simulink library "SUB_L4_Task_10ms"  (R2018a)
settings: Solver=VariableStepAuto  StartTime=0.0  StopTime=10.0  RelTol=1e-3
libraries: EmE_MBD_Blockset x75, simulink x11, SUB_L4_Task_10ms_SUB_APTC x1, SUB_L4_Task_10ms_SUB_BRKPEDARB x1, SUB_L4_Task_10ms_SUB_FAULT_MANAGER x1, SUB_L4_Task_10ms_SUB_STATE_CONTROL x1, SUB_L4_Task_10ms_SUB_STEERCTRL x1, simulink_need_slupdate x1
(part 1 of 2)
settings Model: Creator=Chris.Balton  LastModifiedBy=Gavin.Coelho

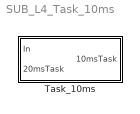
== system SUB_L4_Task_10ms ==
  Task_10ms : Subsystem  TreatAsAtomicUnit=on  SystemSampleTime=0.01

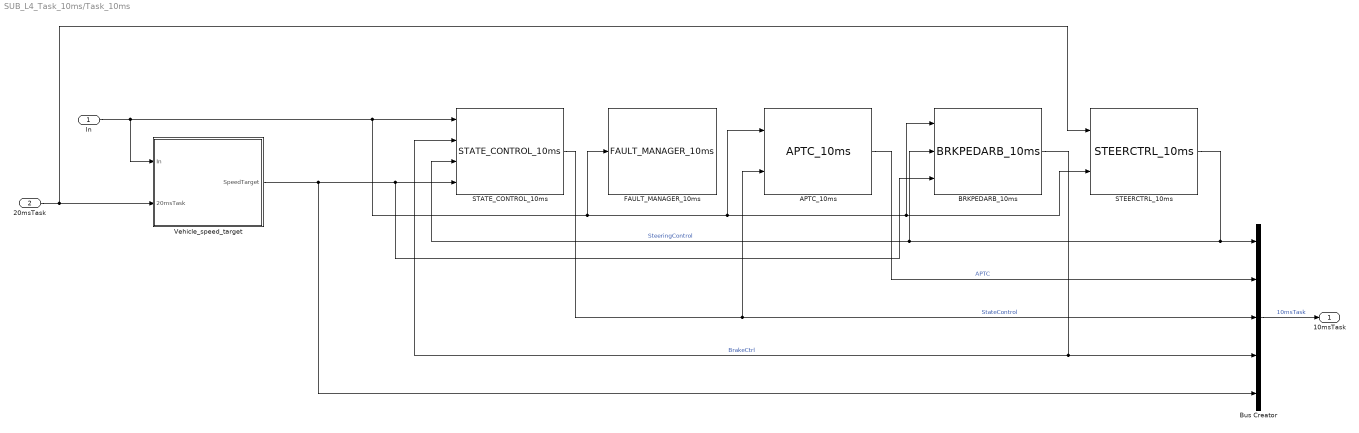
== system SUB_L4_Task_10ms/Task_10ms ==
  In : Inport
  20msTask : Inport  Port=2
  APTC_10ms : SUB_L4_Task_10ms_SUB_APTC/APTC_10ms
  BRKPEDARB_10ms : SUB_L4_Task_10ms_SUB_BRKPEDARB/BRKPEDARB_10ms
  Bus Creator : BusCreator  Inputs=5
  FAULT_MANAGER_10ms : SUB_L4_Task_10ms_SUB_FAULT_MANAGER/FAULT_MANAGER_10ms
  STATE_CONTROL_10ms : SUB_L4_Task_10ms_SUB_STATE_CONTROL/STATE_CONTROL_10ms
  STEERCTRL_10ms : SUB_L4_Task_10ms_SUB_STEERCTRL/STEERCTRL_10ms
  Vehicle_speed_target : Subsystem
  10msTask : Outport
  wires:
  Vehicle_speed_target/1(SpeedTarget) -> BRKPEDARB_10ms/3, STATE_CONTROL_10ms/4, Bus Creator/5
  20msTask/1 -> Vehicle_speed_target/2(20msTask), STEERCTRL_10ms/1
  BRKPEDARB_10ms/1 -> Bus Creator/4, STATE_CONTROL_10ms/2  "BrakeCtrl"
  STATE_CONTROL_10ms/1 -> APTC_10ms/2, Bus Creator/3  "StateControl"
  STEERCTRL_10ms/1 -> BRKPEDARB_10ms/2, STATE_CONTROL_10ms/3, Bus Creator/1  "SteeringControl"
  Bus Creator/1 -> 10msTask/1  "10msTask"
  APTC_10ms/1 -> Bus Creator/2  "APTC"
  In/1 -> Vehicle_speed_target/1(In), STATE_CONTROL_10ms/1, FAULT_MANAGER_10ms/1, APTC_10ms/1, STEERCTRL_10ms/2, BRKPEDARB_10ms/1

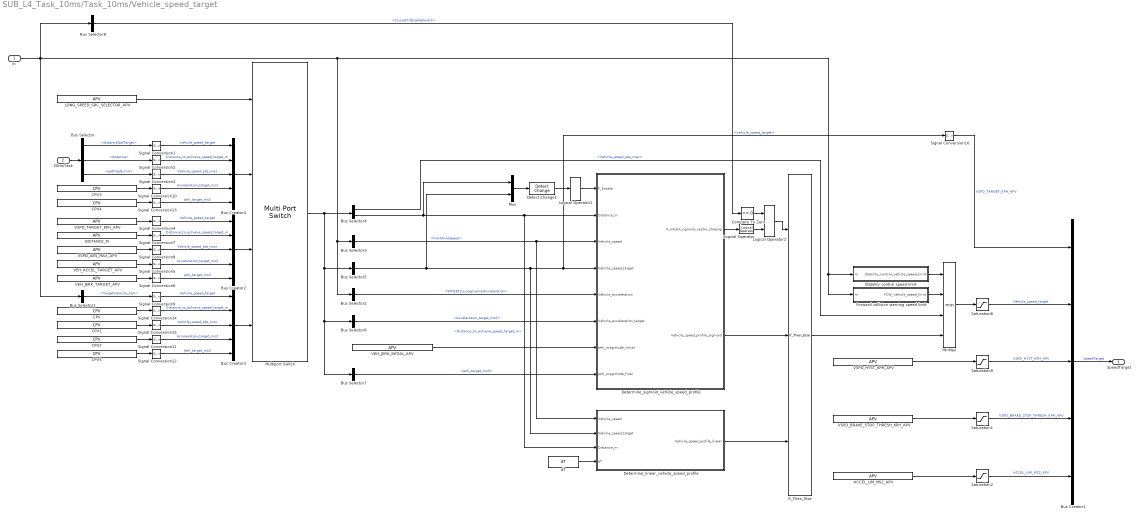
== system SUB_L4_Task_10ms/Task_10ms/Vehicle_speed_target ==
  In : Inport
  20msTask : Inport  Port=2
  ACCEL_LIM_MS2_APV : EmE_MBD_Blockset/Sources/APV  conval=-5
      settings: SourceProductName=PACCAR EmE MBD Blockset
  Bus Creator{1..4} (4 alike) : BusCreator  Inputs=5
  Bus Selector : BusSelector  OutputSignals=mapping.distanceSpdTarget,mapping.distance,mapping.pathSpdLimit
  Bus Selector1 : BusSelector  OutputSignals=PIC_Bus.TargetVelocity_kph
  Bus Selector2 : BusSelector  OutputSignals=CAN.VDC2_0B.SPN1810_LongitudinalAcceleration
  Bus Selector3 : BusSelector  OutputSignals=CAN.EBC2_0B.FrontAxleSpeed
  Bus Selector4 : BusSelector  OutputSignals=Vehicle_speed_abs_max,Distance_to_achieve_speed_target_m
  Bus Selector5 : BusSelector  OutputSignals=Vehicle_speed_target
  Bus Selector6 : BusSelector  OutputSignals=Acceleration_target_ms2
  Bus Selector7 : BusSelector  OutputSignals=Jerk_target_ms3
  Bus Selector8 : BusSelector  OutputSignals=CAN.CCVS_31.CruiseCtrlEnableSwitch
  CPV{,2..4} (4 alike) : EmE_MBD_Blockset/Sources/CPV  conval=0
      settings: SourceProductName=PACCAR EmE MBD Blockset
  CPV1 : EmE_MBD_Blockset/Sources/CPV  conval=255
      settings: SourceProductName=PACCAR EmE MBD Blockset
  CPV5 : EmE_MBD_Blockset/Sources/CPV  conval=0.5
      settings: SourceProductName=PACCAR EmE MBD Blockset
  Compare To Zero : simulink/Logic and Bit Operations/Compare To Zero  relop===  OutDataTypeStr=boolean
  DISTANCE_M : EmE_MBD_Blockset/Sources/APV  conval=DISTANCE_M
      settings: SourceProductName=PACCAR EmE MBD Blockset
  Detect Change1 : simulink/Logic and Bit Operations/Detect Change  vinit=0  InputProcessing=Inherited  OutDataTypeStr=boolean
      settings: AttributesFormatString=IC: %<vinit>
  Determine_linear_vehicle_speed_profile : Subsystem
  Determine_sigmoid_vehicle_speed_profile : Subsystem
  Forward collision warning speed limit : Subsystem
  If_Then_Else : EmE_MBD_Blockset/Signal Routing/If_Then_Else
      settings: SourceProductName=PACCAR EmE MBD Blockset
  LONG_SPEED_SRC_SELECTOR_APV : EmE_MBD_Blockset/Sources/APV  conval=LONG_SPEED_SRC_SELECTOR_APV
      settings: SourceProductName=PACCAR EmE MBD Blockset
  Logical Operator : EmE_MBD_Blockset/Logic and Bit Operations/Logical Operator  Operator=NOT  Inputs=2
      settings: SourceProductName=PACCAR EmE MBD Blockset
  Logical Operator1 : EmE_MBD_Blockset/Logic and Bit Operations/Logical Operator  Operator=OR  Inputs=1
      settings: SourceProductName=PACCAR EmE MBD Blockset
  Logical Operator2 : EmE_MBD_Blockset/Logic and Bit Operations/Logical Operator  Operator=AND  Inputs=2
      settings: SourceProductName=PACCAR EmE MBD Blockset
  MinMax : MinMax  Inputs=4  InputSameDT=on
  Multiport Switch : MultiPortSwitch  DataPortOrder=Specify indices  DataPortIndices={ENUM_LONG_SPEED_DEMAND_SOURCE_T.GPS_PATH,ENUM_LONG_SPEED_DEMAND_SOURCE_T.OVERRIDE,ENUM_LONG_SPEED_DEMAND_SOURCE_T.RW_WAYPOINTS}  DiagnosticForDefault=None
  Mux : Mux  Inputs=2
  Saturation1 : Saturate  UpperLimit=5  LowerLimit=0
      settings: AttributesFormatString=|
      | Min: %<LowerLimit>
      | Max: %<UpperLimit>
  Saturation2 : Saturate  UpperLimit=15.562  LowerLimit=-15.562
      settings: AttributesFormatString=|
      | Min: %<LowerLimit>
      | Max: %<UpperLimit>
  Saturation8 : Saturate  UpperLimit=100  LowerLimit=0
      settings: AttributesFormatString=|
      | Min: %<LowerLimit>
      | Max: %<UpperLimit>
  Saturation9 : Saturate  UpperLimit=5  LowerLimit=0
      settings: AttributesFormatString=|
      | Min: %<LowerLimit>
      | Max: %<UpperLimit>
  Signal Conversion{1..16} (16 alike) : SignalConversion  OverrideOpt=off
  Stability control speed limit : Subsystem
  VEH_ACCEL_TARGET_APV : EmE_MBD_Blockset/Sources/APV  conval=-0.5
      settings: SourceProductName=PACCAR EmE MBD Blockset
  VEH_JERK_INITIAL_APV : EmE_MBD_Blockset/Sources/APV  conval=0.4
      settings: SourceProductName=PACCAR EmE MBD Blockset
  VEH_JERK_TARGET_APV : EmE_MBD_Blockset/Sources/APV  conval=0.2
      settings: SourceProductName=PACCAR EmE MBD Blockset
  VSPD_ABS_MAX_APV : EmE_MBD_Blockset/Sources/APV  conval=255
      settings: SourceProductName=PACCAR EmE MBD Blockset
  VSPD_BRAKE_STOP_THRESH_KPH_APV : EmE_MBD_Blockset/Sources/APV  conval=2
      settings: SourceProductName=PACCAR EmE MBD Blockset
  VSPD_HYST_KPH_APV : EmE_MBD_Blockset/Sources/APV  conval=1
      settings: SourceProductName=PACCAR EmE MBD Blockset
  VSPD_TARGET_KPH_APV : EmE_MBD_Blockset/Sources/APV  conval=VSPD_TARGET_KPH_APV
      settings: SourceProductName=PACCAR EmE MBD Blockset
  dT : EmE_MBD_Blockset/Sources/dT
      settings: SourceProductName=PACCAR EmE MBD Blockset
  SpeedTarget : Outport
  wires:
  Signal Conversion16/1 -> Bus Creator1/1  "VSPD_TARGET_KPH_APV"
  Compare To Zero/1 -> Logical Operator2/1
  Bus Selector8/1 -> Compare To Zero/1  "<CruiseCtrlEnableSwitch>"
  Logical Operator2/1 -> If_Then_Else/1
  VEH_JERK_INITIAL_APV/1 -> Determine_sigmoid_vehicle_speed_profile/7(Jerk_magnitude_initial)
  Bus Selector7/1 -> Determine_sigmoid_vehicle_speed_profile/8(Jerk_magnitude_final)  "<Jerk_target_ms3>"
  CPV5/1 -> Signal Conversion12/1
  Signal Conversion12/1 -> Bus Creator3/5  "Jerk_target_ms3"
  Signal Conversion11/1 -> Bus Creator3/4  "Acceleration_target_ms2"
  Signal Conversion9/1 -> Bus Creator3/1  "Vehicle_speed_target"
  Signal Conversion14/1 -> Bus Creator3/2  "Distance_to_achieve_speed_target_m"
  Signal Conversion15/1 -> Bus Creator3/3  "Vehicle_speed_abs_max"
  Bus Creator3/1 -> Multiport Switch/4
  VEH_JERK_TARGET_APV/1 -> Signal Conversion6/1
  VEH_ACCEL_TARGET_APV/1 -> Signal Conversion5/1
  Bus Creator2/1 -> Multiport Switch/3
  Signal Conversion8/1 -> Bus Creator2/3  "Vehicle_speed_abs_max"
  Signal Conversion7/1 -> Bus Creator2/2  "Distance_to_achieve_speed_target_m"
  Signal Conversion4/1 -> Bus Creator2/1  "Vehicle_speed_target"
  Signal Conversion5/1 -> Bus Creator2/4  "Acceleration_target_ms2"
  Signal Conversion6/1 -> Bus Creator2/5  "Jerk_target_ms3"
  Signal Conversion13/1 -> Bus Creator4/5  "Jerk_target_ms3"
  CPV4/1 -> Signal Conversion13/1
  Determine_sigmoid_vehicle_speed_profile/2(Vehicle_speed_profile_sigmoid) -> If_Then_Else/2
  Bus Selector5/1 -> Mux/2, Determine_sigmoid_vehicle_speed_profile/4(Vehicle_speed_target), Signal Conversion16/1, Determine_linear_vehicle_speed_profile/2(Vehicle_speed_target)  "<Vehicle_speed_target>"
  Mux/1 -> Detect Change1/1
  Detect Change1/1 -> Logical Operator1/1
  Forward collision warning speed limit/1(FCW_vehicle_speed_limit) -> MinMax/2
  Bus Selector4/1 -> MinMax/3  "<Vehicle_speed_abs_max>"
  CPV3/1 -> Signal Conversion10/1
  CPV2/1 -> Signal Conversion11/1
  Signal Conversion10/1 -> Bus Creator4/4  "Acceleration_target_ms2"
  Signal Conversion1/1 -> Bus Creator4/1  "Vehicle_speed_target"
  Signal Conversion2/1 -> Bus Creator4/2  "Distance_to_achieve_speed_target_m"
  Signal Conversion3/1 -> Bus Creator4/3  "Vehicle_speed_abs_max"
  Multiport Switch/1 -> Bus Selector4/1, Bus Selector5/1, Bus Selector6/1, Bus Selector7/1
  CPV1/1 -> Signal Conversion15/1
  CPV/1 -> Signal Conversion14/1
  VSPD_ABS_MAX_APV/1 -> Signal Conversion8/1
  Bus Selector/3 -> Signal Conversion3/1  "<pathSpdLimit>"
  Bus Selector/1 -> Signal Conversion1/1  "<distanceSpdTarget>"
  DISTANCE_M/1 -> Signal Conversion7/1
  VSPD_TARGET_KPH_APV/1 -> Signal Conversion4/1
  Bus Creator4/1 -> Multiport Switch/2
  If_Then_Else/1 -> MinMax/4
  20msTask/1 -> Bus Selector/1
  Bus Selector/2 -> Signal Conversion2/1  "<distance>"
  Bus Selector6/1 -> Determine_sigmoid_vehicle_speed_profile/6(Vehicle_acceleration_target)  "<Acceleration_target_ms2>"
  Logical Operator/1 -> Logical Operator2/2
  Bus Selector4/2 -> Mux/1, Determine_linear_vehicle_speed_profile/3(Distance_m), Determine_sigmoid_vehicle_speed_profile/2(Distance_m)  "<Distance_to_achieve_speed_target_m>"
  Bus Selector3/1 -> Determine_linear_vehicle_speed_profile/1(Vehicle_speed), Determine_sigmoid_vehicle_speed_profile/3(Vehicle_speed)  "<FrontAxleSpeed>"
  Logical Operator1/1 -> Determine_sigmoid_vehicle_speed_profile/1(F_Enable)
  dT/1 -> Determine_linear_vehicle_speed_profile/4(dT)
  Bus Selector2/1 -> Determine_sigmoid_vehicle_speed_profile/5(Vehicle_acceleration)  "<SPN1810_LongitudinalAcceleration>"
  Determine_sigmoid_vehicle_speed_profile/1(F_Inhibit_sigmoid_vector_shaping) -> Logical Operator/1
  Determine_linear_vehicle_speed_profile/1(Vehicle_speed_profile_linear) -> If_Then_Else/3
  Bus Creator1/1 -> SpeedTarget/1  "SpeedTarget"
  Saturation9/1 -> Bus Creator1/3  "VSPD_HYST_KPH_APV"
  Saturation2/1 -> Bus Creator1/5  "ACCEL_LIM_MS2_APV"
  Bus Selector1/1 -> Signal Conversion9/1  "<TargetVelocity_kph>"
  ACCEL_LIM_MS2_APV/1 -> Saturation2/1
  VSPD_BRAKE_STOP_THRESH_KPH_APV/1 -> Saturation1/1
  MinMax/1 -> Saturation8/1
  Saturation1/1 -> Bus Creator1/4  "VSPD_BRAKE_STOP_THRESH_KPH_APV"
  LONG_SPEED_SRC_SELECTOR_APV/1 -> Multiport Switch/1
  Stability control speed limit/1(Stability_control_vehicle_speed_limit) -> MinMax/1
  Saturation8/1 -> Bus Creator1/2  "Vehicle_speed_target"
  VSPD_HYST_KPH_APV/1 -> Saturation9/1
  In/1 -> Bus Selector8/1, Forward collision warning speed limit/1(In), Stability control speed limit/1(In), Bus Selector3/1, Bus Selector2/1, Bus Selector1/1

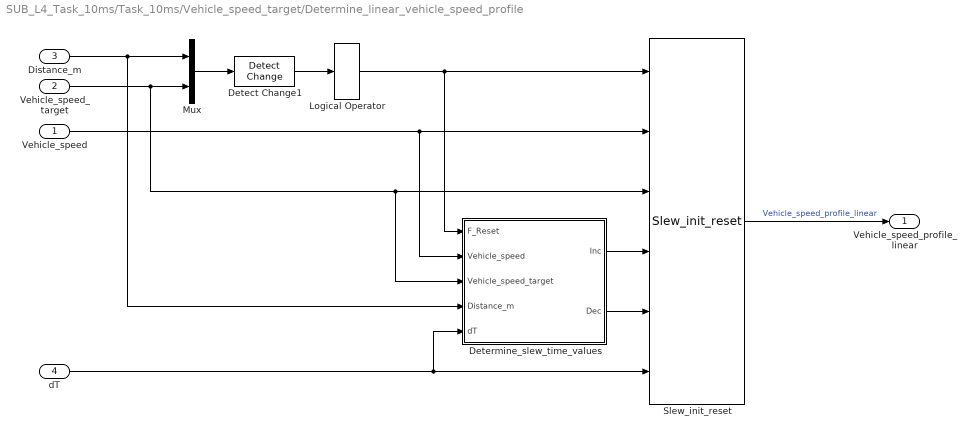
== system SUB_L4_Task_10ms/Task_10ms/Vehicle_speed_target/Determine_linear_vehicle_speed_profile ==
  Vehicle_speed : Inport
  Vehicle_speed_target : Inport  Port=2
  Distance_m : Inport  Port=3
  dT : Inport  Port=4
  Detect Change1 : simulink/Logic and Bit Operations/Detect Change  vinit=0  InputProcessing=Inherited  OutDataTypeStr=boolean
      settings: AttributesFormatString=IC: %<vinit>
  Determine_slew_time_values : Subsystem
  Logical Operator : EmE_MBD_Blockset/Logic and Bit Operations/Logical Operator  Operator=OR  Inputs=1
      settings: SourceProductName=PACCAR EmE MBD Blockset
  Mux : Mux  Inputs=2
  Slew_init_reset : EmE_MBD_Blockset/Math Operators/Slew_init_reset
      settings: SourceProductName=PACCAR EmE MBD Blockset
  Vehicle_speed_profile_linear : Outport  OutputWhenDisabled=reset
  wires:
  Determine_slew_time_values/2(Dec) -> Slew_init_reset/5
  Determine_slew_time_values/1(Inc) -> Slew_init_reset/4
  Vehicle_speed/1 -> Slew_init_reset/2, Determine_slew_time_values/2(Vehicle_speed)
  Distance_m/1 -> Mux/1, Determine_slew_time_values/4(Distance_m)
  Vehicle_speed_target/1 -> Mux/2, Slew_init_reset/3, Determine_slew_time_values/3(Vehicle_speed_target)
  Logical Operator/1 -> Slew_init_reset/1, Determine_slew_time_values/1(F_Reset)
  Mux/1 -> Detect Change1/1
  Detect Change1/1 -> Logical Operator/1
  Slew_init_reset/1 -> Vehicle_speed_profile_linear/1  "Vehicle_speed_profile_linear"
  dT/1 -> Determine_slew_time_values/5(dT), Slew_init_reset/6

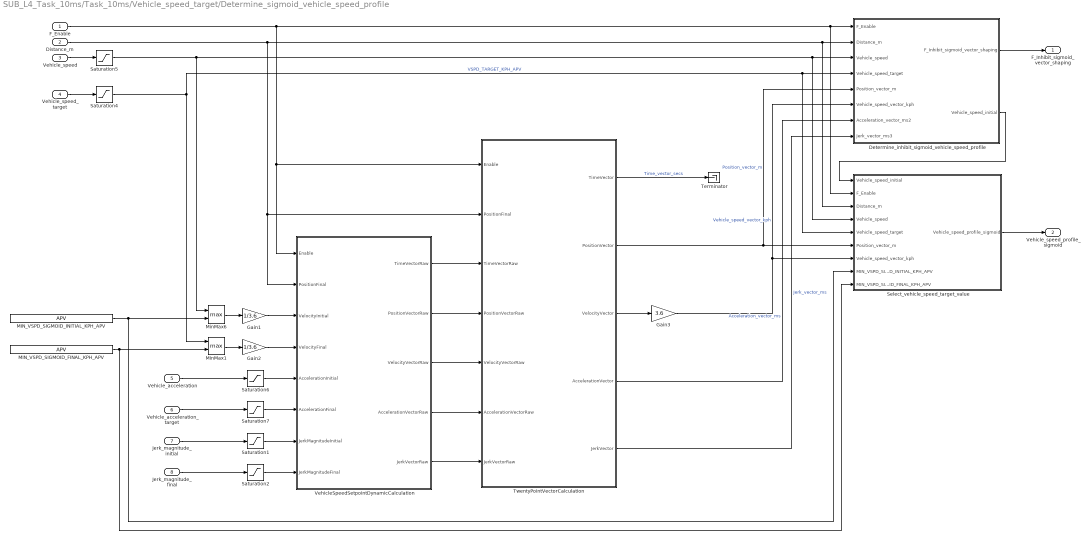
== system SUB_L4_Task_10ms/Task_10ms/Vehicle_speed_target/Determine_sigmoid_vehicle_speed_profile ==
  F_Enable : Inport
  Distance_m : Inport  Port=2
  Vehicle_speed : Inport  Port=3
  Vehicle_speed_target : Inport  Port=4
  Vehicle_acceleration : Inport  Port=5
  Vehicle_acceleration_target : Inport  Port=6
  Jerk_magnitude_initial : Inport  Port=7
  Jerk_magnitude_final : Inport  Port=8
  Determine_inhibit_sigmoid_vehicle_speed_profile : Subsystem
  Gain1 : Gain  Gain=1/3.6
  Gain2 : Gain  Gain=1/3.6
  Gain3 : Gain  Gain=3.6
  MIN_VSPD_SIGMOID_FINAL_KPH_APV : EmE_MBD_Blockset/Sources/APV  conval=0
      settings: SourceProductName=PACCAR EmE MBD Blockset
  MIN_VSPD_SIGMOID_INITIAL_KPH_APV : EmE_MBD_Blockset/Sources/APV  conval=5
      settings: SourceProductName=PACCAR EmE MBD Blockset
  MinMax1 : MinMax  Function=max  Inputs=2  InputSameDT=on
  MinMax6 : MinMax  Function=max  Inputs=2  InputSameDT=on
  Saturation1 : Saturate  UpperLimit=10  LowerLimit=0.001
      settings: AttributesFormatString=|
      | Min: %<LowerLimit>
      | Max: %<UpperLimit>
  Saturation2 : Saturate  UpperLimit=10  LowerLimit=0.001
      settings: AttributesFormatString=|
      | Min: %<LowerLimit>
      | Max: %<UpperLimit>
  Saturation4 : Saturate  UpperLimit=255  LowerLimit=0
      settings: AttributesFormatString=|
      | Min: %<LowerLimit>
      | Max: %<UpperLimit>
  Saturation5 : Saturate  UpperLimit=255  LowerLimit=0
      settings: AttributesFormatString=|
      | Min: %<LowerLimit>
      | Max: %<UpperLimit>
  Saturation6 : Saturate  UpperLimit=15.562  LowerLimit=-15.562
      settings: AttributesFormatString=|
      | Min: %<LowerLimit>
      | Max: %<UpperLimit>
  Saturation7 : Saturate  UpperLimit=15.562  LowerLimit=-15.562
      settings: AttributesFormatString=|
      | Min: %<LowerLimit>
      | Max: %<UpperLimit>
  Select_vehicle_speed_target_value : Subsystem
  Terminator : Terminator
  TwentyPointVectorCalculation : Stateflow chart  TreatAsAtomicUnit=on
  VehicleSpeedSetpointDynamicCalculation : Stateflow chart  TreatAsAtomicUnit=on
  F_Inhibit_sigmoid_vector_shaping : Outport  LibraryBlock=EmE_MBD_Blockset/Sinks/Out  OutputWhenDisabled=reset
  Vehicle_speed_profile_sigmoid : Outport  Port=2
  wires:
  F_Enable/1 -> VehicleSpeedSetpointDynamicCalculation/1(Enable), TwentyPointVectorCalculation/1(Enable), Select_vehicle_speed_target_value/2(F_Enable), Determine_inhibit_sigmoid_vehicle_speed_profile/1(F_Enable)
  Distance_m/1 -> VehicleSpeedSetpointDynamicCalculation/2(PositionFinal), TwentyPointVectorCalculation/2(PositionFinal), Select_vehicle_speed_target_value/3(Distance_m), Determine_inhibit_sigmoid_vehicle_speed_profile/2(Distance_m)
  Gain2/1 -> VehicleSpeedSetpointDynamicCalculation/4(VelocityFinal)
  Gain1/1 -> VehicleSpeedSetpointDynamicCalculation/3(VelocityInitial)
  Vehicle_acceleration/1 -> Saturation6/1
  Gain3/1 -> Determine_inhibit_sigmoid_vehicle_speed_profile/6(Vehicle_speed_vector_kph), Select_vehicle_speed_target_value/7(Vehicle_speed_vector_kph)  "Vehicle_speed_vector_kph"
  Vehicle_acceleration_target/1 -> Saturation7/1
  Determine_inhibit_sigmoid_vehicle_speed_profile/1(F_Inhibit_sigmoid_vector_shaping) -> F_Inhibit_sigmoid_vector_shaping/1
  Vehicle_speed/1 -> Saturation5/1
  Select_vehicle_speed_target_value/1(Vehicle_speed_profile_sigmoid) -> Vehicle_speed_profile_sigmoid/1
  VehicleSpeedSetpointDynamicCalculation/5(JerkVectorRaw) -> TwentyPointVectorCalculation/7(JerkVectorRaw)
  TwentyPointVectorCalculation/1(TimeVector) -> Terminator/1  "Time_vector_secs"
  TwentyPointVectorCalculation/3(VelocityVector) -> Gain3/1
  VehicleSpeedSetpointDynamicCalculation/4(AccelerationVectorRaw) -> TwentyPointVectorCalculation/6(AccelerationVectorRaw)
  TwentyPointVectorCalculation/4(AccelerationVector) -> Determine_inhibit_sigmoid_vehicle_speed_profile/7(Acceleration_vector_ms2)  "Acceleration_vector_ms"
  VehicleSpeedSetpointDynamicCalculation/2(PositionVectorRaw) -> TwentyPointVectorCalculation/4(PositionVectorRaw)
  TwentyPointVectorCalculation/5(JerkVector) -> Determine_inhibit_sigmoid_vehicle_speed_profile/8(Jerk_vector_ms3)  "Jerk_vector_ms"
  VehicleSpeedSetpointDynamicCalculation/1(TimeVectorRaw) -> TwentyPointVectorCalculation/3(TimeVectorRaw)
  TwentyPointVectorCalculation/2(PositionVector) -> Determine_inhibit_sigmoid_vehicle_speed_profile/5(Position_vector_m), Select_vehicle_speed_target_value/6(Position_vector_m)  "Position_vector_m"
  VehicleSpeedSetpointDynamicCalculation/3(VelocityVectorRaw) -> TwentyPointVectorCalculation/5(VelocityVectorRaw)
  Jerk_magnitude_initial/1 -> Saturation1/1
  Jerk_magnitude_final/1 -> Saturation2/1
  MIN_VSPD_SIGMOID_INITIAL_KPH_APV/1 -> MinMax6/2, Select_vehicle_speed_target_value/8(MIN_VSPD_SIGMOID_INITIAL_KPH_APV)
  MIN_VSPD_SIGMOID_FINAL_KPH_APV/1 -> MinMax1/2, Select_vehicle_speed_target_value/9(MIN_VSPD_SIGMOID_FINAL_KPH_APV)
  MinMax1/1 -> Gain2/1
  MinMax6/1 -> Gain1/1
  Determine_inhibit_sigmoid_vehicle_speed_profile/2(Vehicle_speed_initial) -> Select_vehicle_speed_target_value/1(Vehicle_speed_initial)
  Saturation4/1 -> MinMax1/1, Select_vehicle_speed_target_value/5(Vehicle_speed_target), Determine_inhibit_sigmoid_vehicle_speed_profile/4(Vehicle_speed_target)  "VSPD_TARGET_KPH_APV"
  Saturation5/1 -> MinMax6/1, Select_vehicle_speed_target_value/4(Vehicle_speed), Determine_inhibit_sigmoid_vehicle_speed_profile/3(Vehicle_speed)
  Vehicle_speed_target/1 -> Saturation4/1
  Saturation6/1 -> VehicleSpeedSetpointDynamicCalculation/5(AccelerationInitial)
  Saturation7/1 -> VehicleSpeedSetpointDynamicCalculation/6(AccelerationFinal)
  Saturation1/1 -> VehicleSpeedSetpointDynamicCalculation/7(JerkMagnitudeInitial)
  Saturation2/1 -> VehicleSpeedSetpointDynamicCalculation/8(JerkMagnitudeFinal)

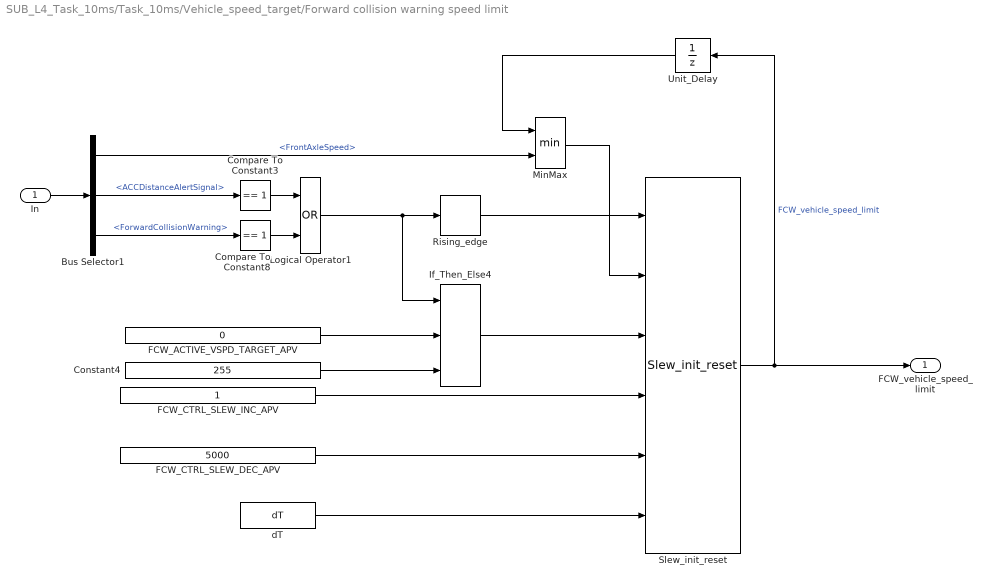
== system SUB_L4_Task_10ms/Task_10ms/Vehicle_speed_target/Forward collision warning speed limit ==
  In : Inport
  Bus Selector1 : BusSelector  OutputSignals=CAN.EBC2_0B.FrontAxleSpeed,CAN.ACC1_2A.ACCDistanceAlertSignal,CAN.ACC1_2A.ForwardCollisionWarning
  Compare To Constant3 : simulink/Logic and Bit Operations/Compare To Constant  relop===  const=1  OutDataTypeStr=boolean
  Compare To Constant8 : simulink/Logic and Bit Operations/Compare To Constant  relop===  const=1  OutDataTypeStr=boolean
  Constant4 : Constant  Value=255
  FCW_ACTIVE_VSPD_TARGET_APV : Constant  Value=0
  FCW_CTRL_SLEW_DEC_APV : Constant  Value=5000
  FCW_CTRL_SLEW_INC_APV : Constant
  If_Then_Else4 : EmE_MBD_Blockset/Signal Routing/If_Then_Else
      settings: SourceProductName=PACCAR EmE MBD Blockset
  Logical Operator1 : Logic  Operator=OR  OutDataTypeStr=boolean
  MinMax : MinMax  Inputs=2  InputSameDT=on
  Rising_edge : EmE_MBD_Blockset/Discontinuities/Rising_edge  initact=off
      settings: AttributesFormatString=Action on IC: %<initact>  SourceProductName=PACCAR EmE MBD Blockset
  Slew_init_reset : EmE_MBD_Blockset/Math Operators/Slew_init_reset
      settings: SourceProductName=PACCAR EmE MBD Blockset
  Unit_Delay : UnitDelay  SampleTime=-1
      settings: AttributesFormatString=IC: %<vinit>
  dT : EmE_MBD_Blockset/Sources/dT
      settings: SourceProductName=PACCAR EmE MBD Blockset
  FCW_vehicle_speed_limit : Outport
  wires:
  MinMax/1 -> Slew_init_reset/2
  FCW_CTRL_SLEW_INC_APV/1 -> Slew_init_reset/4
  FCW_ACTIVE_VSPD_TARGET_APV/1 -> If_Then_Else4/2
  FCW_CTRL_SLEW_DEC_APV/1 -> Slew_init_reset/5
  Slew_init_reset/1 -> Unit_Delay/1, FCW_vehicle_speed_limit/1  "FCW_vehicle_speed_limit"
  Bus Selector1/1 -> MinMax/2  "<FrontAxleSpeed>"
  Constant4/1 -> If_Then_Else4/3
  dT/1 -> Slew_init_reset/6
  Logical Operator1/1 -> Rising_edge/1, If_Then_Else4/1
  If_Then_Else4/1 -> Slew_init_reset/3
  Unit_Delay/1 -> MinMax/1
  Rising_edge/1 -> Slew_init_reset/1
  Bus Selector1/3 -> Compare To Constant8/1  "<ForwardCollisionWarning>"
  Compare To Constant8/1 -> Logical Operator1/2
  Bus Selector1/2 -> Compare To Constant3/1  "<ACCDistanceAlertSignal>"
  Compare To Constant3/1 -> Logical Operator1/1
  In/1 -> Bus Selector1/1

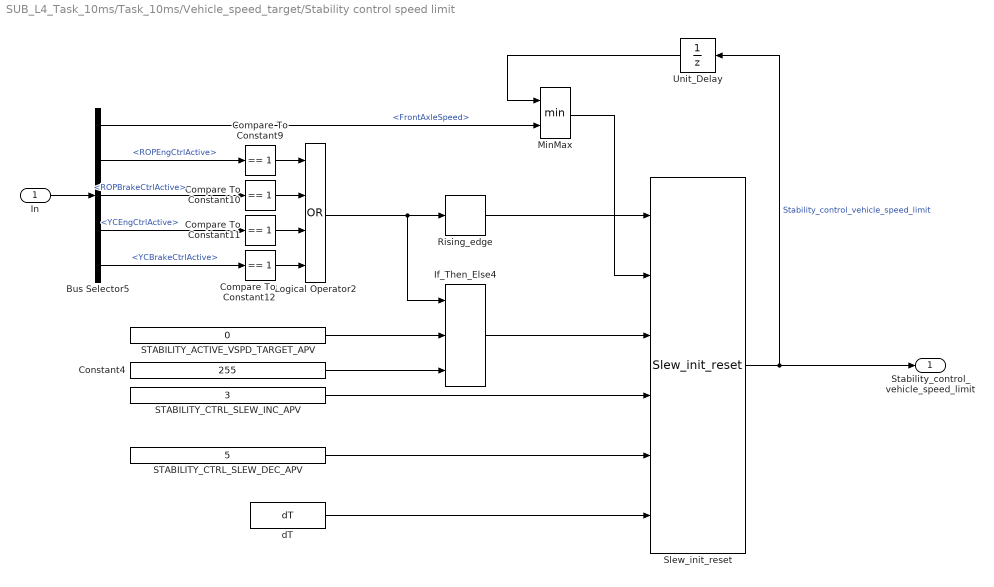
== system SUB_L4_Task_10ms/Task_10ms/Vehicle_speed_target/Stability control speed limit ==
  In : Inport
  Bus Selector5 : BusSelector  OutputSignals=CAN.EBC2_0B.FrontAxleSpeed,CAN.VDC1_0B.ROPEngCtrlActive,CAN.VDC1_0B.ROPBrakeCtrlActive,CAN.VDC1_0B.YCEngCtrlActive,CAN.VDC1_0B.YCBrakeCtrlActive
  Compare To Constant{9..12} (4 alike) : simulink/Logic and Bit Operations/Compare To Constant  relop===  const=1  OutDataTypeStr=boolean
  Constant4 : Constant  Value=255
  If_Then_Else4 : EmE_MBD_Blockset/Signal Routing/If_Then_Else
      settings: SourceProductName=PACCAR EmE MBD Blockset
  Logical Operator2 : Logic  Operator=OR  Inputs=4  OutDataTypeStr=boolean
  MinMax : MinMax  Inputs=2  InputSameDT=on
  Rising_edge : EmE_MBD_Blockset/Discontinuities/Rising_edge  initact=off
      settings: AttributesFormatString=Action on IC: %<initact>  SourceProductName=PACCAR EmE MBD Blockset
  STABILITY_ACTIVE_VSPD_TARGET_APV : Constant  Value=0
  STABILITY_CTRL_SLEW_DEC_APV : Constant  Value=5
  STABILITY_CTRL_SLEW_INC_APV : Constant  Value=3
  Slew_init_reset : EmE_MBD_Blockset/Math Operators/Slew_init_reset
      settings: SourceProductName=PACCAR EmE MBD Blockset
  Unit_Delay : UnitDelay  SampleTime=-1
      settings: AttributesFormatString=IC: %<vinit>
  dT : EmE_MBD_Blockset/Sources/dT
      settings: SourceProductName=PACCAR EmE MBD Blockset
  Stability_control_vehicle_speed_limit : Outport
  wires:
  Unit_Delay/1 -> MinMax/1
  Bus Selector5/1 -> MinMax/2  "<FrontAxleSpeed>"
  MinMax/1 -> Slew_init_reset/2
  Rising_edge/1 -> Slew_init_reset/1
  Slew_init_reset/1 -> Unit_Delay/1, Stability_control_vehicle_speed_limit/1  "Stability_control_vehicle_speed_limit"
  Logical Operator2/1 -> Rising_edge/1, If_Then_Else4/1
  Bus Selector5/3 -> Compare To Constant10/1  "<ROPBrakeCtrlActive>"
  In/1 -> Bus Selector5/1
  If_Then_Else4/1 -> Slew_init_reset/3
  STABILITY_ACTIVE_VSPD_TARGET_APV/1 -> If_Then_Else4/2
  STABILITY_CTRL_SLEW_DEC_APV/1 -> Slew_init_reset/5
  STABILITY_CTRL_SLEW_INC_APV/1 -> Slew_init_reset/4
  Constant4/1 -> If_Then_Else4/3
  dT/1 -> Slew_init_reset/6
  Compare To Constant11/1 -> Logical Operator2/3
  Compare To Constant9/1 -> Logical Operator2/1
  Compare To Constant12/1 -> Logical Operator2/4
  Compare To Constant10/1 -> Logical Operator2/2
  Bus Selector5/5 -> Compare To Constant12/1  "<YCBrakeCtrlActive>"
  Bus Selector5/2 -> Compare To Constant9/1  "<ROPEngCtrlActive>"
  Bus Selector5/4 -> Compare To Constant11/1  "<YCEngCtrlActive>"

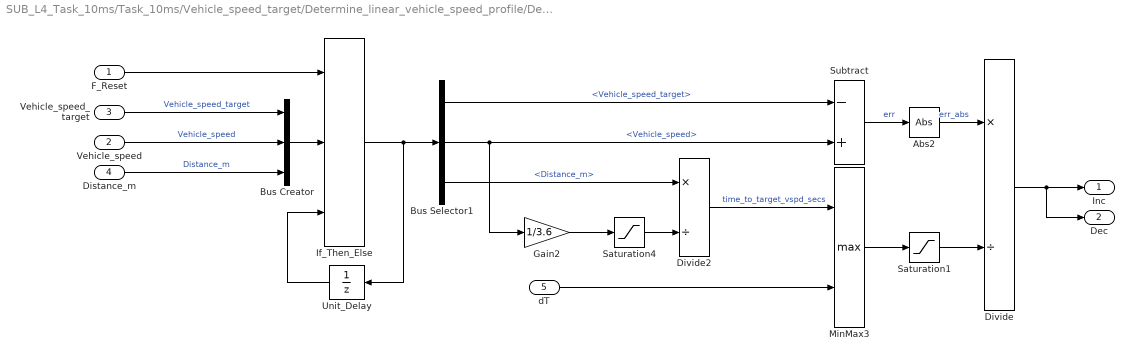
== system SUB_L4_Task_10ms/Task_10ms/Vehicle_speed_target/Determine_linear_vehicle_speed_profile/Determine_slew_time_values ==
  F_Reset : Inport
  Vehicle_speed : Inport  Port=2
  Vehicle_speed_target : Inport  Port=3
  Distance_m : Inport  Port=4
  dT : Inport  Port=5
  Abs2 : EmE_MBD_Blockset/Math Operators/Abs
      settings: SourceProductName=PACCAR EmE MBD Blockset
  Bus Creator : BusCreator  Inputs=3
  Bus Selector1 : BusSelector  OutputSignals=Vehicle_speed_target,Vehicle_speed,Distance_m
  Divide : Product  Inputs=*/  InputSameDT=on
  Divide2 : Product  Inputs=*/  InputSameDT=on
  Gain2 : Gain  Gain=1/3.6
  If_Then_Else : EmE_MBD_Blockset/Signal Routing/If_Then_Else
      settings: SourceProductName=PACCAR EmE MBD Blockset
  MinMax3 : MinMax  Function=max  Inputs=2  InputSameDT=on
  Saturation1 : Saturate  UpperLimit=Inf  LowerLimit=0.001
      settings: AttributesFormatString=|
      | Min: %<LowerLimit>
      | Max: %<UpperLimit>
  Saturation4 : Saturate  UpperLimit=255  LowerLimit=0.001
      settings: AttributesFormatString=|
      | Min: %<LowerLimit>
      | Max: %<UpperLimit>
  Subtract : Sum  Inputs=-+  InputSameDT=on
  Unit_Delay : UnitDelay  SampleTime=-1
      settings: AttributesFormatString=IC: %<vinit>
  Inc : Outport
  Dec : Outport  Port=2
  wires:
  F_Reset/1 -> If_Then_Else/1
  Vehicle_speed/1 -> Bus Creator/2  "Vehicle_speed"
  Vehicle_speed_target/1 -> Bus Creator/1  "Vehicle_speed_target"
  Distance_m/1 -> Bus Creator/3  "Distance_m"
  Unit_Delay/1 -> If_Then_Else/3
  If_Then_Else/1 -> Bus Selector1/1, Unit_Delay/1
  Bus Creator/1 -> If_Then_Else/2
  Saturation1/1 -> Divide/2
  Divide/1 -> Inc/1, Dec/1
  Abs2/1 -> Divide/1  "err_abs"
  MinMax3/1 -> Saturation1/1
  Saturation4/1 -> Divide2/2
  dT/1 -> MinMax3/2
  Bus Selector1/1 -> Subtract/1  "<Vehicle_speed_target>"
  Divide2/1 -> MinMax3/1  "time_to_target_vspd_secs"
  Gain2/1 -> Saturation4/1
  Subtract/1 -> Abs2/1  "err"
  Bus Selector1/3 -> Divide2/1  "<Distance_m>"
  Bus Selector1/2 -> Subtract/2, Gain2/1  "<Vehicle_speed>"

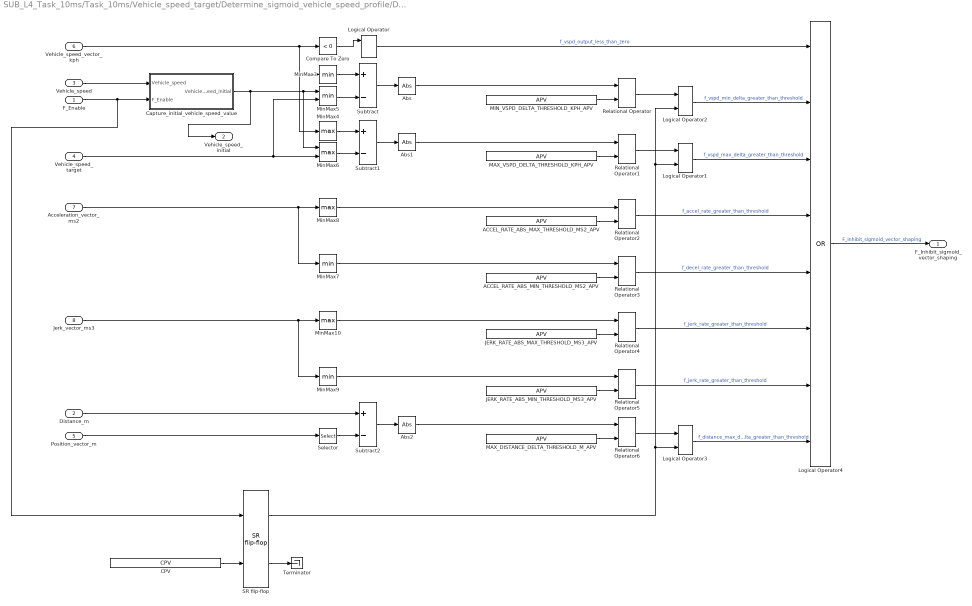
== system SUB_L4_Task_10ms/Task_10ms/Vehicle_speed_target/Determine_sigmoid_vehicle_speed_profile/Determine_inhibit_sigmoid_vehicle_speed_profile ==
  F_Enable : Inport
  Distance_m : Inport  Port=2
  Vehicle_speed : Inport  Port=3
  Vehicle_speed_target : Inport  Port=4
  Position_vector_m : Inport  Port=5
  Vehicle_speed_vector_kph : Inport  Port=6
  Acceleration_vector_ms2 : Inport  Port=7
  Jerk_vector_ms3 : Inport  Port=8
  ACCEL_RATE_ABS_MAX_THRESHOLD_MS2_APV : EmE_MBD_Blockset/Sources/APV  conval=5
      settings: SourceProductName=PACCAR EmE MBD Blockset
  ACCEL_RATE_ABS_MIN_THRESHOLD_MS2_APV : EmE_MBD_Blockset/Sources/APV  conval=-5
      settings: SourceProductName=PACCAR EmE MBD Blockset
  Abs : EmE_MBD_Blockset/Math Operators/Abs
      settings: SourceProductName=PACCAR EmE MBD Blockset
  Abs1 : EmE_MBD_Blockset/Math Operators/Abs
      settings: SourceProductName=PACCAR EmE MBD Blockset
  Abs2 : EmE_MBD_Blockset/Math Operators/Abs
      settings: SourceProductName=PACCAR EmE MBD Blockset
  CPV : EmE_MBD_Blockset/Sources/CPV  conval=false
      settings: SourceProductName=PACCAR EmE MBD Blockset
  Capture_initial_vehicle_speed_value : Subsystem
  Compare To Zero : simulink/Logic and Bit Operations/Compare To Zero  relop=<  OutDataTypeStr=boolean
  JERK_RATE_ABS_MAX_THRESHOLD_MS3_APV : EmE_MBD_Blockset/Sources/APV  conval=5
      settings: SourceProductName=PACCAR EmE MBD Blockset
  JERK_RATE_ABS_MIN_THRESHOLD_MS3_APV : EmE_MBD_Blockset/Sources/APV  conval=-5
      settings: SourceProductName=PACCAR EmE MBD Blockset
  Logical Operator : EmE_MBD_Blockset/Logic and Bit Operations/Logical Operator  Operator=OR  Inputs=1
      settings: SourceProductName=PACCAR EmE MBD Blockset
  Logical Operator1 : EmE_MBD_Blockset/Logic and Bit Operations/Logical Operator  Operator=AND  Inputs=2
      settings: SourceProductName=PACCAR EmE MBD Blockset
  Logical Operator2 : EmE_MBD_Blockset/Logic and Bit Operations/Logical Operator  Operator=AND  Inputs=2
      settings: SourceProductName=PACCAR EmE MBD Blockset
  Logical Operator3 : EmE_MBD_Blockset/Logic and Bit Operations/Logical Operator  Operator=AND  Inputs=2
      settings: SourceProductName=PACCAR EmE MBD Blockset
  Logical Operator4 : Logic  Operator=OR  Inputs=8  AllPortsSameDT=off  OutDataTypeStr=boolean
  MAX_DISTANCE_DELTA_THRESHOLD_M_APV : EmE_MBD_Blockset/Sources/APV  conval=0.5
      settings: SourceProductName=PACCAR EmE MBD Blockset
  MAX_VSPD_DELTA_THRESHOLD_KPH_APV : EmE_MBD_Blockset/Sources/APV  conval=5
      settings: SourceProductName=PACCAR EmE MBD Blockset
  MIN_VSPD_DELTA_THRESHOLD_KPH_APV : EmE_MBD_Blockset/Sources/APV  conval=5
      settings: SourceProductName=PACCAR EmE MBD Blockset
  MinMax10 : MinMax  Function=max  InputSameDT=on
  MinMax3 : MinMax  InputSameDT=on
  MinMax4 : MinMax  Function=max  InputSameDT=on
  MinMax5 : MinMax  Inputs=2  InputSameDT=on
  MinMax6 : MinMax  Function=max  Inputs=2  InputSameDT=on
  MinMax7 : MinMax  InputSameDT=on
  MinMax8 : MinMax  Function=max  InputSameDT=on
  MinMax9 : MinMax  InputSameDT=on
  Relational Operator{,1..2,4,6} (5 alike) : EmE_MBD_Blockset/Logic and Bit Operations/Relational Operator  func=>
      settings: SourceProductName=PACCAR EmE MBD Blockset
  Relational Operator3 : EmE_MBD_Blockset/Logic and Bit Operations/Relational Operator  func=<
      settings: SourceProductName=PACCAR EmE MBD Blockset
  Relational Operator5 : EmE_MBD_Blockset/Logic and Bit Operations/Relational Operator  func=<
      settings: SourceProductName=PACCAR EmE MBD Blockset
  SR flip-flop : EmE_MBD_Blockset/Logic and Bit Operations/SR flip-flop
      settings: SourceProductName=PACCAR EmE MBD Blockset
  Selector : Selector  InputPortWidth=33  IndexOptions=Index vector (dialog)  Indices=33  OutputSizes=1
  Subtract : Sum  Inputs=+-  InputSameDT=on
  Subtract1 : Sum  Inputs=+-  InputSameDT=on
  Subtract2 : Sum  Inputs=+-  InputSameDT=on
  Terminator : Terminator
  F_Inhibit_sigmoid_vector_shaping : Outport  LibraryBlock=EmE_MBD_Blockset/Sinks/Out  OutputWhenDisabled=reset
  Vehicle_speed_initial : Outport  Port=2
  wires:
  Compare To Zero/1 -> Logical Operator/1
  F_Enable/1 -> SR flip-flop/1, Capture_initial_vehicle_speed_value/2(F_Enable)
  ACCEL_RATE_ABS_MIN_THRESHOLD_MS2_APV/1 -> Relational Operator3/2
  Logical Operator4/1 -> F_Inhibit_sigmoid_vector_shaping/1  "F_Inhibit_sigmoid_vector_shaping"
  CPV/1 -> SR flip-flop/2
  Relational Operator4/1 -> Logical Operator4/6  "f_jerk_rate_greater_than_threshold"
  SR flip-flop/2 -> Terminator/1
  MinMax7/1 -> Relational Operator3/1
  SR flip-flop/1 -> Logical Operator3/2, Logical Operator1/2, Logical Operator2/2
  MinMax3/1 -> Subtract/1
  Relational Operator3/1 -> Logical Operator4/5  "f_decel_rate_greater_than_threshold"
  Relational Operator2/1 -> Logical Operator4/4  "f_accel_rate_greater_than_threshold"
  Vehicle_speed_vector_kph/1 -> MinMax4/1, MinMax3/1, Compare To Zero/1
  Acceleration_vector_ms2/1 -> MinMax7/1, MinMax8/1
  JERK_RATE_ABS_MAX_THRESHOLD_MS3_APV/1 -> Relational Operator4/2
  Relational Operator/1 -> Logical Operator2/1
  MinMax8/1 -> Relational Operator2/1
  ACCEL_RATE_ABS_MAX_THRESHOLD_MS2_APV/1 -> Relational Operator2/2
  MinMax10/1 -> Relational Operator4/1
  Relational Operator5/1 -> Logical Operator4/7  "f_jerk_rate_greater_than_threshold"
  Logical Operator1/1 -> Logical Operator4/3  "f_vspd_max_delta_greater_than_threshold"
  Abs/1 -> Relational Operator/1
  Abs1/1 -> Relational Operator1/1
  Jerk_vector_ms3/1 -> MinMax9/1, MinMax10/1
  MIN_VSPD_DELTA_THRESHOLD_KPH_APV/1 -> Relational Operator/2
  MinMax4/1 -> Subtract1/1
  Logical Operator/1 -> Logical Operator4/1  "f_vspd_output_less_than_zero"
  JERK_RATE_ABS_MIN_THRESHOLD_MS3_APV/1 -> Relational Operator5/2
  MinMax9/1 -> Relational Operator5/1
  Logical Operator2/1 -> Logical Operator4/2  "f_vspd_min_delta_greater_than_threshold"
  MAX_VSPD_DELTA_THRESHOLD_KPH_APV/1 -> Relational Operator1/2
  Relational Operator1/1 -> Logical Operator1/1
  Subtract1/1 -> Abs1/1
  Subtract/1 -> Abs/1
  MinMax5/1 -> Subtract/2
  MinMax6/1 -> Subtract1/2
  Vehicle_speed_target/1 -> MinMax5/2, MinMax6/2
  Capture_initial_vehicle_speed_value/1(Vehicle_speed_initial) -> Vehicle_speed_initial/1, MinMax6/1, MinMax5/1
  Vehicle_speed/1 -> Capture_initial_vehicle_speed_value/1(Vehicle_speed)
  MAX_DISTANCE_DELTA_THRESHOLD_M_APV/1 -> Relational Operator6/2
  Abs2/1 -> Relational Operator6/1
  Subtract2/1 -> Abs2/1
  Distance_m/1 -> Subtract2/1
  Logical Operator3/1 -> Logical Operator4/8  "f_distance_max_delta_greater_than_threshold"
  Selector/1 -> Subtract2/2
  Position_vector_m/1 -> Selector/1
  Relational Operator6/1 -> Logical Operator3/1

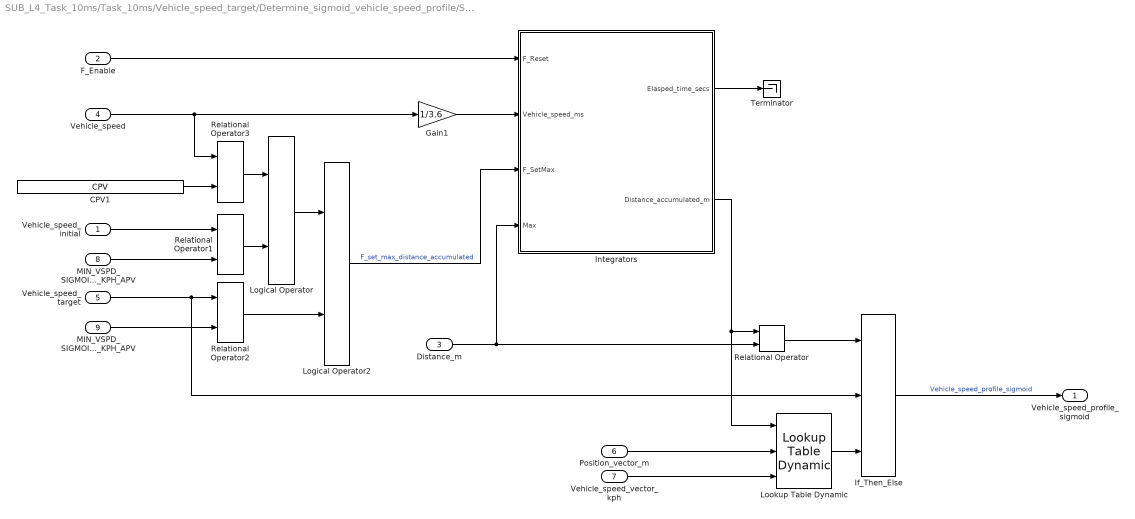
== system SUB_L4_Task_10ms/Task_10ms/Vehicle_speed_target/Determine_sigmoid_vehicle_speed_profile/Select_vehicle_speed_target_value ==
  Vehicle_speed_initial : Inport
  F_Enable : Inport  Port=2
  Distance_m : Inport  Port=3
  Vehicle_speed : Inport  Port=4
  Vehicle_speed_target : Inport  Port=5
  Position_vector_m : Inport  Port=6
  Vehicle_speed_vector_kph : Inport  Port=7
  MIN_VSPD_SIGMOID_INITIAL_KPH_APV : Inport  Port=8
  MIN_VSPD_SIGMOID_FINAL_KPH_APV : Inport  Port=9
  CPV1 : EmE_MBD_Blockset/Sources/CPV  conval=0.1
      settings: SourceProductName=PACCAR EmE MBD Blockset
  Gain1 : Gain  Gain=1/3.6
  If_Then_Else : EmE_MBD_Blockset/Signal Routing/If_Then_Else
      settings: SourceProductName=PACCAR EmE MBD Blockset
  Integrators : Subsystem
  Logical Operator : EmE_MBD_Blockset/Logic and Bit Operations/Logical Operator  Operator=OR  Inputs=2
      settings: SourceProductName=PACCAR EmE MBD Blockset
  Logical Operator2 : EmE_MBD_Blockset/Logic and Bit Operations/Logical Operator  Operator=AND  Inputs=2
      settings: SourceProductName=PACCAR EmE MBD Blockset
  Lookup Table Dynamic : simulink/Lookup Tables/Lookup Table Dynamic  LookUpMeth=Interpolation-Use End Values  OutDataType=fixdt('double')  OutScaling=[]  OutputDataTypeScalingMode=Specify via dialog  OutDataTypeStr=double  DoSatur=off
      settings: SourceProductName=Simulink
  Relational Operator : EmE_MBD_Blockset/Logic and Bit Operations/Relational Operator  func===
      settings: SourceProductName=PACCAR EmE MBD Blockset
  Relational Operator1 : EmE_MBD_Blockset/Logic and Bit Operations/Relational Operator  func=<
      settings: SourceProductName=PACCAR EmE MBD Blockset
  Relational Operator2 : EmE_MBD_Blockset/Logic and Bit Operations/Relational Operator  func=<
      settings: SourceProductName=PACCAR EmE MBD Blockset
  Relational Operator3 : EmE_MBD_Blockset/Logic and Bit Operations/Relational Operator  func=<
      settings: SourceProductName=PACCAR EmE MBD Blockset
  Terminator : Terminator
  Vehicle_speed_profile_sigmoid : Outport
  wires:
  Vehicle_speed_target/1 -> If_Then_Else/2, Relational Operator2/1
  If_Then_Else/1 -> Vehicle_speed_profile_sigmoid/1  "Vehicle_speed_profile_sigmoid"
  Distance_m/1 -> Relational Operator/2, Integrators/4(Max)
  Vehicle_speed/1 -> Relational Operator3/1, Gain1/1
  Position_vector_m/1 -> Lookup Table Dynamic/2
  Integrators/1(Elasped_time_secs) -> Terminator/1
  Vehicle_speed_vector_kph/1 -> Lookup Table Dynamic/3
  Lookup Table Dynamic/1 -> If_Then_Else/3
  F_Enable/1 -> Integrators/1(F_Reset)
  Vehicle_speed_initial/1 -> Relational Operator1/1
  Relational Operator2/1 -> Logical Operator2/2
  MIN_VSPD_SIGMOID_INITIAL_KPH_APV/1 -> Relational Operator1/2
  MIN_VSPD_SIGMOID_FINAL_KPH_APV/1 -> Relational Operator2/2
  Integrators/2(Distance_accumulated_m) -> Lookup Table Dynamic/1, Relational Operator/1
  Gain1/1 -> Integrators/2(Vehicle_speed_ms)
  Relational Operator/1 -> If_Then_Else/1
  Relational Operator3/1 -> Logical Operator/1
  Logical Operator/1 -> Logical Operator2/1
  Relational Operator1/1 -> Logical Operator/2
  CPV1/1 -> Relational Operator3/2
  Logical Operator2/1 -> Integrators/3(F_SetMax)  "F_set_max_distance_accumulated"

== system SUB_L4_Task_10ms/Task_10ms/Vehicle_speed_target/Determine_sigmoid_vehicle_speed_profile/Determine_inhibit_sigmoid_vehicle_speed_profile/Capture_initial_vehicle_speed_value ==
  Vehicle_speed : Inport
  F_Enable : Inport  Port=2
  If_Then_Else : EmE_MBD_Blockset/Signal Routing/If_Then_Else
      settings: SourceProductName=PACCAR EmE MBD Blockset
  Unit_Delay : UnitDelay  SampleTime=-1
      settings: AttributesFormatString=IC: %<vinit>
  Vehicle_speed_initial : Outport
  wires:
  If_Then_Else/1 -> Unit_Delay/1, Vehicle_speed_initial/1  "Vehicle_speed_initial"
  F_Enable/1 -> If_Then_Else/1
  Unit_Delay/1 -> If_Then_Else/3
  Vehicle_speed/1 -> If_Then_Else/2

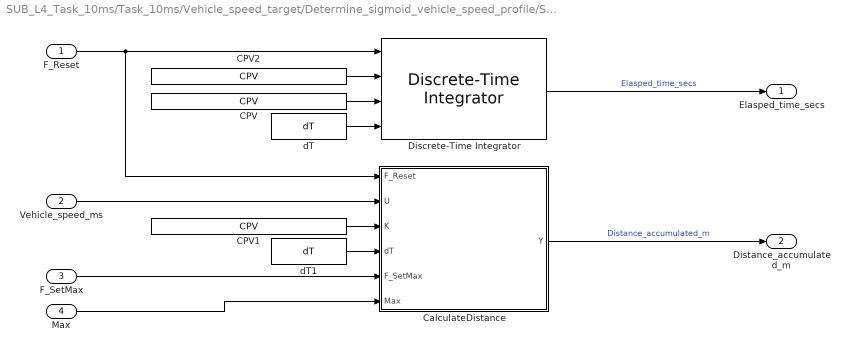
== system SUB_L4_Task_10ms/Task_10ms/Vehicle_speed_target/Determine_sigmoid_vehicle_speed_profile/Select_vehicle_speed_target_value/Integrators ==
  F_Reset : Inport
  Vehicle_speed_ms : Inport  Port=2
  F_SetMax : Inport  Port=3
  Max : Inport  Port=4
  CPV : EmE_MBD_Blockset/Sources/CPV  conval=1
      settings: SourceProductName=PACCAR EmE MBD Blockset
  CPV1 : EmE_MBD_Blockset/Sources/CPV  conval=1
      settings: SourceProductName=PACCAR EmE MBD Blockset
  CPV2 : EmE_MBD_Blockset/Sources/CPV  conval=1
      settings: SourceProductName=PACCAR EmE MBD Blockset
  CalculateDistance : Subsystem
  Discrete-Time Integrator : EmE_MBD_Blockset/Discrete/Discrete-Time Integrator  integrator_method_sel=Backward Euler
      settings: AttributesFormatString=%<integrator_method_sel>  SourceProductName=PACCAR EmE MBD Blockset
  dT : EmE_MBD_Blockset/Sources/dT
      settings: SourceProductName=PACCAR EmE MBD Blockset
  dT1 : EmE_MBD_Blockset/Sources/dT
      settings: SourceProductName=PACCAR EmE MBD Blockset
  Elasped_time_secs : Outport
  Distance_accumulated_m : Outport  Port=2
  wires:
  dT/1 -> Discrete-Time Integrator/4
  CalculateDistance/1(Y) -> Distance_accumulated_m/1  "Distance_accumulated_m"
  CPV/1 -> Discrete-Time Integrator/3
  Vehicle_speed_ms/1 -> CalculateDistance/2(U)
  F_Reset/1 -> CalculateDistance/1(F_Reset), Discrete-Time Integrator/1
  Discrete-Time Integrator/1 -> Elasped_time_secs/1  "Elasped_time_secs"
  dT1/1 -> CalculateDistance/4(dT)
  CPV1/1 -> CalculateDistance/3(K)
  CPV2/1 -> Discrete-Time Integrator/2
  Max/1 -> CalculateDistance/6(Max)
  F_SetMax/1 -> CalculateDistance/5(F_SetMax)

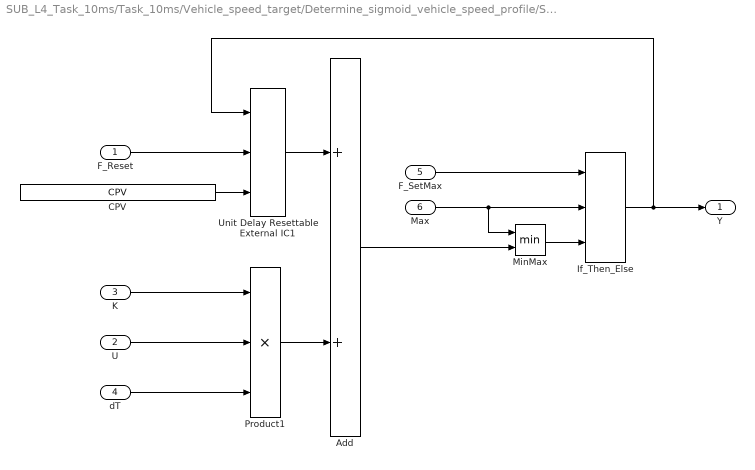
== system SUB_L4_Task_10ms/Task_10ms/Vehicle_speed_target/Determine_sigmoid_vehicle_speed_profile/Select_vehicle_speed_target_value/Integrators/CalculateDistance ==
  F_Reset : Inport
  U : Inport  Port=2
  K : Inport  Port=3
  dT : Inport  Port=4
  F_SetMax : Inport  Port=5
  Max : Inport  Port=6
  Add : Sum  InputSameDT=on
  CPV : EmE_MBD_Blockset/Sources/CPV  conval=0
      settings: SourceProductName=PACCAR EmE MBD Blockset
  If_Then_Else : EmE_MBD_Blockset/Signal Routing/If_Then_Else
      settings: SourceProductName=PACCAR EmE MBD Blockset
  MinMax : MinMax  Inputs=2  InputSameDT=on
  Product1 : Product  Inputs=3  InputSameDT=on
  Unit Delay Resettable External IC1 : simulink_need_slupdate/Unit Delay Resettable External IC  tsamp=-1
      settings: SourceProductName=Simulink  SourceProductBaseCode=SL
  Y : Outport  OutputWhenDisabled=reset  InitialOutput=0
  wires:
  U/1 -> Product1/2
  K/1 -> Product1/1
  dT/1 -> Product1/3
  Max/1 -> MinMax/1, If_Then_Else/2
  F_SetMax/1 -> If_Then_Else/1
  MinMax/1 -> If_Then_Else/3
  If_Then_Else/1 -> Unit Delay Resettable External IC1/1, Y/1
  Unit Delay Resettable External IC1/1 -> Add/1
  CPV/1 -> Unit Delay Resettable External IC1/3
  Add/1 -> MinMax/2
  Product1/1 -> Add/2
  F_Reset/1 -> Unit Delay Resettable External IC1/2

== stateflow chart SUB_L4_Task_10ms/Task_10ms/Vehicle_speed_target/Determine_sigmoid_vehicle_speed_profile/TwentyPointVectorCalculation ==
  (default) -> (junction 85)
  (junction 85) -> (junction 86) [order 1] : [Enable]
  (junction 85) -> (junction 87) [order 2]
  (junction 86) -> (junction 21) : {TimeVector(1) = TimeVectorRaw(1);
      | JerkVector(1) = JerkVectorRaw(1);
      | AccelerationVector(1) = AccelerationVectorRaw(1);
      | VelocityVector(1) = VelocityVectorRaw(1);
      | PositionVector(1) = PositionVectorRaw(1);
      |
      | TimeIncrement = (TimeVectorRaw(2) - TimeVectorRaw(1)) / 10;
      | i = 2;}
  (junction 21) -> (junction 19) [order 1] : [i <= 10]
  (junction 19) -> (junction 22) : {TimeVector(i) = TimeVector(i-1) + TimeIncrement;
      | DeltaTime = TimeVector(i) - TimeVectorRaw(1);
      | JerkVector(i) = JerkVectorRaw(1);
      | AccelerationVector(i) = AccelerationVectorRaw(1) + JerkVectorRaw(1) * DeltaTime;
      | VelocityVector(i) = VelocityVectorRaw(1) + AccelerationVectorRaw(1) * DeltaTime + 0.5 * JerkVectorRaw(1) * DeltaTime^2;
      | PositionVector(i) = PositionVectorRaw(1) + VelocityVectorRaw(1) * DeltaTime + 0.5 * AccelerationVectorRaw(1) * DeltaTime^2 + (JerkVectorRaw(1) / 6) * DeltaTime^3;
      | PositionVector(i) = max(PositionVector(i-1) + 0.0001, PositionVector(i));}
  (junction 22) -> (junction 21) : {i = i + 1;}
  (junction 21) -> (junction 129) [order 2] : {TimeVector(11) = TimeVectorRaw(2);
      | JerkVector(11) = JerkVectorRaw(2);
      | AccelerationVector(11) = AccelerationVectorRaw(2);
      | VelocityVector(11) = VelocityVectorRaw(2);
      | PositionVector(11) = max(PositionVector(10) + 0.0001, PositionVectorRaw(2));
      |
      | TimeVector(12) = TimeVectorRaw(3);
      | JerkVector(12) = JerkVectorRaw(3);
      | AccelerationVector(12) = AccelerationVectorRaw(3);
      | VelocityVector(12) = VelocityVectorRaw(3);
      | PositionVector(12) = max(PositionVector(11) + 0.0001, PositionVectorRaw(3));
      |
      | TimeIncrement = (TimeVectorRaw(4) - TimeVectorRaw(3)) / 10;
      | i = 13;}
  (junction 129) -> (junction 128) [order 1] : [i <= 21]
  (junction 128) -> (junction 130) : {TimeVector(i) = TimeVector(i-1) + TimeIncrement;
      | DeltaTime = TimeVector(i) - TimeVectorRaw(3);
      | JerkVector(i) = JerkVectorRaw(3);
      | AccelerationVector(i) = AccelerationVectorRaw(3) + JerkVectorRaw(3) * DeltaTime;
      | VelocityVector(i) = VelocityVectorRaw(3) + AccelerationVectorRaw(3) * DeltaTime + 0.5 * JerkVectorRaw(3) * DeltaTime^2;
      | PositionVector(i) = PositionVectorRaw(3) + VelocityVectorRaw(3) * DeltaTime + 0.5 * AccelerationVectorRaw(3) * DeltaTime^2 + (JerkVectorRaw(3) / 6) * DeltaTime^3;
      | PositionVector(i) = max(PositionVector(i-1) + 0.0001, PositionVector(i));}
  (junction 130) -> (junction 129) : {i = i + 1;}
  (junction 129) -> (junction 109) [order 2] : {TimeVector(22) = TimeVectorRaw(4);
      | JerkVector(22) = JerkVectorRaw(4);
      | AccelerationVector(22) = AccelerationVectorRaw(4);
      | VelocityVector(22) = VelocityVectorRaw(4);
      | PositionVector(22) = max(PositionVector(21) + 0.0001, PositionVectorRaw(4));
      |
      | TimeVector(23) = TimeVectorRaw(5);
      | JerkVector(23) = JerkVectorRaw(5);
      | AccelerationVector(23) = AccelerationVectorRaw(5);
      | VelocityVector(23) = VelocityVectorRaw(5);
      | PositionVector(23) = max(PositionVector(22) + 0.0001, PositionVectorRaw(5));
      |
      | TimeIncrement = (TimeVectorRaw(6) - TimeVectorRaw(5)) / 10;
      | i = 24;}
  (junction 109) -> (junction 107) [order 1] : [i <= 32]
  (junction 107) -> (junction 108) : {TimeVector(i) = TimeVector(i-1) + TimeIncrement;
      | DeltaTime = TimeVector(i) - TimeVectorRaw(5);
      | JerkVector(i) = JerkVectorRaw(5);
      | AccelerationVector(i) = AccelerationVectorRaw(5) + JerkVectorRaw(5) * DeltaTime;
      | VelocityVector(i) = VelocityVectorRaw(5) + AccelerationVectorRaw(5) * DeltaTime + 0.5 * JerkVectorRaw(5) * DeltaTime^2;
      | PositionVector(i) = PositionVectorRaw(5) + VelocityVectorRaw(5) * DeltaTime + 0.5 * AccelerationVectorRaw(5) * DeltaTime^2 + (JerkVectorRaw(5) / 6) * DeltaTime^3;
      | PositionVector(i) = max(PositionVector(i-1) + 0.0001, PositionVector(i));}
  (junction 108) -> (junction 109) : {i = i + 1;}
  (junction 109) -> (junction 23) [order 2] : {TimeVector(33) = TimeVectorRaw(6);
      | JerkVector(33) = JerkVectorRaw(6);
      | AccelerationVector(33) = AccelerationVectorRaw(6);
      | VelocityVector(33) = VelocityVectorRaw(6);
      | PositionVector(33) = max(PositionVector(32) + 0.0001, PositionVectorRaw(6));}
  (junction 23) -> (junction 87)
  (junction 87) -> (junction 92)
  data: TimeVector output size=33 =[0:0.001:0.032]'; PositionVector output size=33 =[0:0.001:0.032]'; VelocityVector output size=33 =zeros(33,1); AccelerationVector output size=33 =zeros(33,1); JerkVector output size=33 =zeros(33,1); Enable input; PositionFinal input; TimeVectorRaw input; PositionVectorRaw input; VelocityVectorRaw input; AccelerationVectorRaw input; JerkVectorRaw input; i local uint8; DeltaTime local double; TimeIncrement local double
